simulink model "attitude_filter_wrapper"  (R2023a)
settings: configuration reference "configuration_filter" (kept outside this file)
undefined symbols (not defined in the file): DiscIntNeverNeededParam, Eul_rad, filt, mode, rot_K_est_OB_B_radDs, rot_K_meas_IB_B_radDs, sfor_est_B_mDs, sfor_meas_B_mDs2, sim, x_est
libraries: lib_kinematics x5
settings Model: Creator=FC_dev1  LastModifiedBy=FC_dev1
settings ConfigSetRef: SourceName=configuration_filter  SourceLocation=Base Workspace

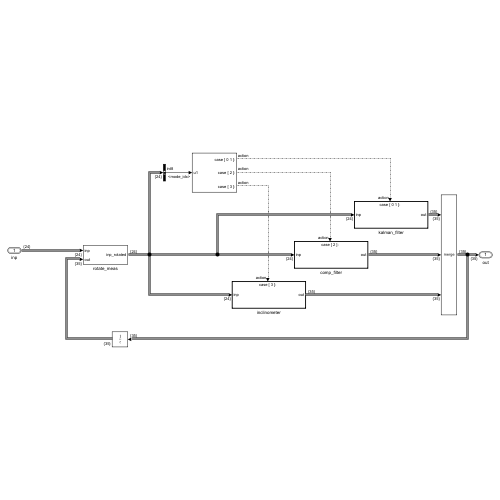
[thumbnail: Simulink's stored preview of the top-level diagram]
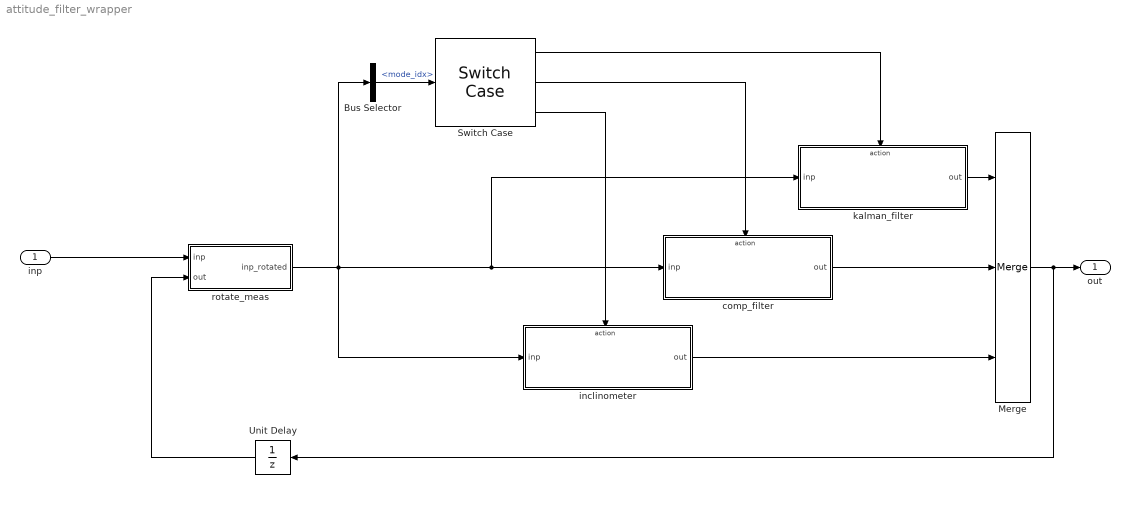
== system attitude_filter_wrapper ==
  inp : Inport  OutDataTypeStr=Bus: inp_Bus
  Bus Selector : BusSelector  OutputSignals=mode_idx
  Merge : Merge  Inputs=3
  Switch Case : SwitchCase  CaseConditions={[filt.modes.kalman_filter, filt.modes.dead_reckoning], filt.modes.comp_filter, filt.modes.inclinometer}  ShowDefaultCase=off
  Unit Delay : UnitDelay  SampleTime=-1  HasFrameUpgradeWarning=on
  comp_filter : Subsystem
  inclinometer : Subsystem
  kalman_filter : Subsystem
  rotate_meas : Subsystem
  out : Outport  OutDataTypeStr=Bus: out_Bus
  wires:
  inp/1 -> rotate_meas/1(inp)
  comp_filter/1(out) -> Merge/2
  Bus Selector/1 -> Switch Case/1  "<mode_idx>"
  Switch Case/1 -> kalman_filter/Action
  Switch Case/2 -> comp_filter/Action
  kalman_filter/1(out) -> Merge/1
  Merge/1 -> Unit Delay/1, out/1
  inclinometer/1(out) -> Merge/3
  Switch Case/3 -> inclinometer/Action
  Unit Delay/1 -> rotate_meas/2(out)
  rotate_meas/1(inp_rotated) -> inclinometer/1(inp), comp_filter/1(inp), kalman_filter/1(inp), Bus Selector/1

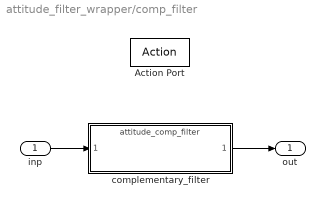
== system attitude_filter_wrapper/comp_filter ==
  inp : Inport  OutDataTypeStr=Bus: inp_Bus
  Action Port : ActionPort  InitializeStates=reset  ActionPortLabel=case [ 2 ]:
  complementary_filter : ModelReference  ModelNameDialog=attitude_comp_filter.slx  SimulationMode=Normal  ModelReferenceVersion=1.231
  out : Outport  OutDataTypeStr=Bus: out_Bus
  wires:
  inp/1 -> complementary_filter/1
  complementary_filter/1 -> out/1

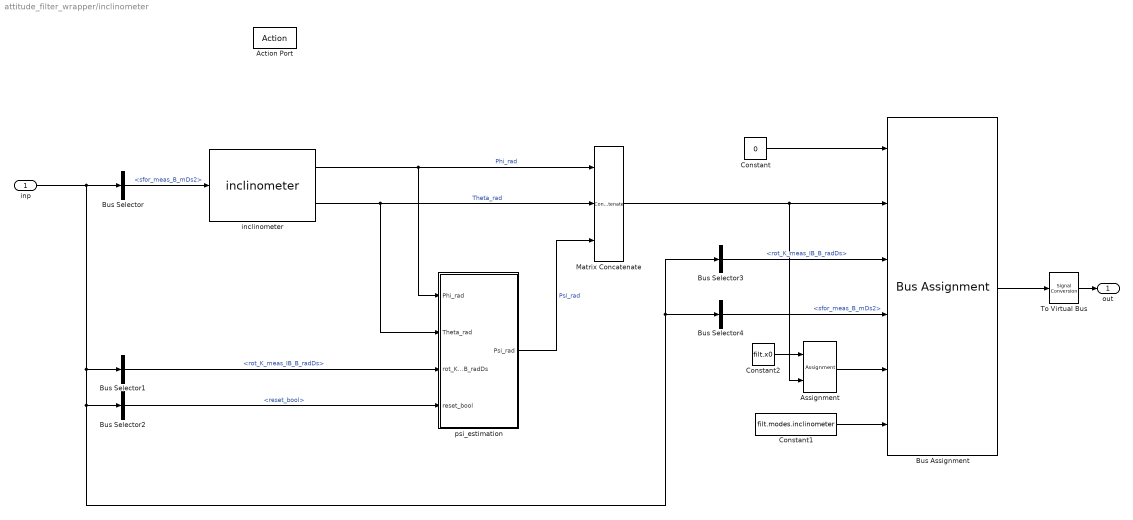
== system attitude_filter_wrapper/inclinometer ==
  inp : Inport  OutDataTypeStr=Bus: inp_Bus
  Action Port : ActionPort  InitializeStates=reset  ActionPortLabel=case [ 3 ]:
  Assignment : Assignment  NumberOfDimensions=2  DiagnosticForDimensions=Warning  IndexOptions=Index vector (dialog),Index vector (dialog)  Indices=filt.eul_idx,1  OutputSizes=1,1
  Bus Assignment : BusAssignment  AssignedSignals=Eul_rad,rot_K_est_OB_B_radDs,sfor_est_B_mDs,x_est,mode
  Bus Selector : BusSelector  OutputSignals=sfor_meas_B_mDs2
  Bus Selector1 : BusSelector  OutputSignals=rot_K_meas_IB_B_radDs
  Bus Selector2 : BusSelector  OutputSignals=reset_bool
  Bus Selector3 : BusSelector  OutputSignals=rot_K_meas_IB_B_radDs
  Bus Selector4 : BusSelector  OutputSignals=sfor_meas_B_mDs2
  Constant : Constant  Value=0  OutDataTypeStr=Bus: out_Bus
  Constant1 : Constant  Value=filt.modes.inclinometer
  Constant2 : Constant  Value=filt.x0  VectorParams1D=off
  Matrix Concatenate : Concatenate  NumInputs=3  Mode=Multidimensional array
  To Virtual Bus : SignalConversion  ConversionOutput=Virtual bus  OverrideOpt=off
  inclinometer : lib_kinematics/inclinometer  SystemSampleTime=-1  VariantActivationTime=update diagram  Latency=0  AutoFrameSizeCalculation=off
  psi_estimation : Subsystem
  out : Outport  OutDataTypeStr=Bus: out_Bus
  wires:
  inp/1 -> Bus Selector4/1, Bus Selector3/1, Bus Selector2/1, Bus Selector1/1, Bus Selector/1
  Bus Selector/1 -> inclinometer/1  "<sfor_meas_B_mDs2>"
  inclinometer/1 -> psi_estimation/1(Phi_rad), Matrix Concatenate/1  "Phi_rad"
  inclinometer/2 -> psi_estimation/2(Theta_rad), Matrix Concatenate/2  "Theta_rad"
  Bus Selector2/1 -> psi_estimation/4(reset_bool)  "<reset_bool>"
  Bus Selector1/1 -> psi_estimation/3(rot_K_OB_B_radDs)  "<rot_K_meas_IB_B_radDs>"
  Constant/1 -> Bus Assignment/1
  psi_estimation/1(Psi_rad) -> Matrix Concatenate/3  "Psi_rad"
  Matrix Concatenate/1 -> Assignment/2, Bus Assignment/2
  Bus Selector3/1 -> Bus Assignment/3  "<rot_K_meas_IB_B_radDs>"
  Bus Selector4/1 -> Bus Assignment/4  "<sfor_meas_B_mDs2>"
  Bus Assignment/1 -> To Virtual Bus/1
  To Virtual Bus/1 -> out/1
  Constant2/1 -> Assignment/1
  Assignment/1 -> Bus Assignment/5
  Constant1/1 -> Bus Assignment/6

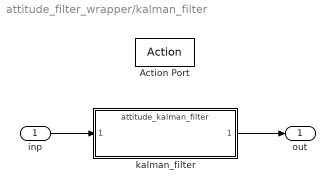
== system attitude_filter_wrapper/kalman_filter ==
  inp : Inport  OutDataTypeStr=Bus: inp_Bus
  Action Port : ActionPort  InitializeStates=reset  ActionPortLabel=case [ 0 1 ]:
  kalman_filter : ModelReference  ModelNameDialog=attitude_kalman_filter.slx  SimulationMode=Normal  ModelReferenceVersion=1.354
  out : Outport  OutDataTypeStr=Bus: out_Bus
  wires:
  inp/1 -> kalman_filter/1
  kalman_filter/1 -> out/1

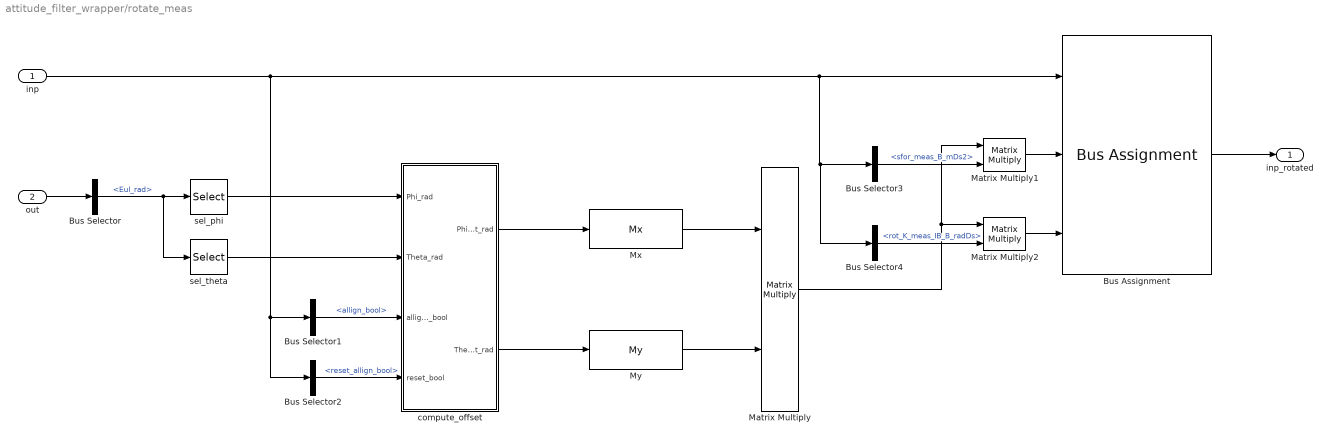
== system attitude_filter_wrapper/rotate_meas ==
  inp : Inport  OutDataTypeStr=Bus: inp_Bus
  out : Inport  Port=2  OutDataTypeStr=Bus: out_Bus
  Bus Assignment : BusAssignment  AssignedSignals=sfor_meas_B_mDs2,rot_K_meas_IB_B_radDs
  Bus Selector : BusSelector  OutputSignals=Eul_rad
  Bus Selector1 : BusSelector  OutputSignals=allign_bool
  Bus Selector2 : BusSelector  OutputSignals=reset_allign_bool
  Bus Selector3 : BusSelector  OutputSignals=sfor_meas_B_mDs2
  Bus Selector4 : BusSelector  OutputSignals=rot_K_meas_IB_B_radDs
  Matrix Multiply : Product  Multiplication=Matrix(*)
  Matrix Multiply1 : Product  Multiplication=Matrix(*)
  Matrix Multiply2 : Product  Multiplication=Matrix(*)
  Mx : lib_kinematics/Mx  SystemSampleTime=-1  VariantActivationTime=update diagram  Latency=0  AutoFrameSizeCalculation=off
  My : lib_kinematics/My  SystemSampleTime=-1  VariantActivationTime=update diagram  Latency=0  AutoFrameSizeCalculation=off
  compute_offset : Subsystem
  sel_phi : Selector  NumberOfDimensions=2  InputPortWidth=3  IndexOptions=Index vector (dialog),Index vector (dialog)  Indices=1,1  OutputSizes=1,1
  sel_theta : Selector  NumberOfDimensions=2  InputPortWidth=3  IndexOptions=Index vector (dialog),Index vector (dialog)  Indices=2,1  OutputSizes=1,1
  inp_rotated : Outport  OutDataTypeStr=Bus: inp_Bus
  wires:
  inp/1 -> Bus Selector2/1, Bus Selector1/1, Bus Selector4/1, Bus Selector3/1, Bus Assignment/1
  out/1 -> Bus Selector/1
  Bus Selector/1 -> sel_theta/1, sel_phi/1  "<Eul_rad>"
  sel_phi/1 -> compute_offset/1(Phi_rad)
  sel_theta/1 -> compute_offset/2(Theta_rad)
  Bus Selector1/1 -> compute_offset/3(allign_bool)  "<allign_bool>"
  Bus Selector2/1 -> compute_offset/4(reset_bool)  "<reset_allign_bool>"
  compute_offset/1(Phi_offset_rad) -> Mx/1
  compute_offset/2(Theta_offset_rad) -> My/1
  Mx/1 -> Matrix Multiply/1
  My/1 -> Matrix Multiply/2
  Bus Assignment/1 -> inp_rotated/1
  Matrix Multiply1/1 -> Bus Assignment/2
  Matrix Multiply/1 -> Matrix Multiply2/1, Matrix Multiply1/1
  Matrix Multiply2/1 -> Bus Assignment/3
  Bus Selector3/1 -> Matrix Multiply1/2  "<sfor_meas_B_mDs2>"
  Bus Selector4/1 -> Matrix Multiply2/2  "<rot_K_meas_IB_B_radDs>"

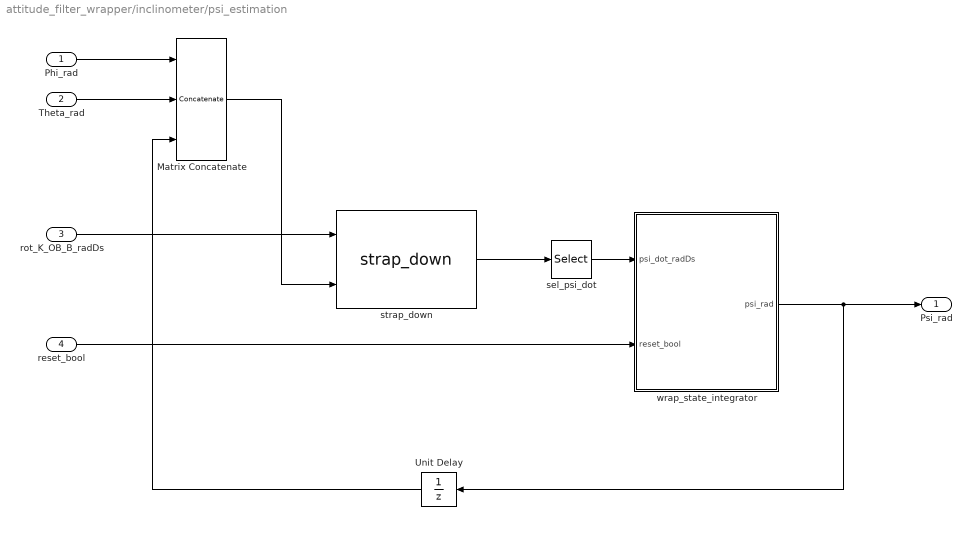
== system attitude_filter_wrapper/inclinometer/psi_estimation ==
  Phi_rad : Inport
  Theta_rad : Inport  Port=2
  rot_K_OB_B_radDs : Inport  Port=3  OutDataTypeStr=single  PortDimensions=[3 1]
  reset_bool : Inport  Port=4
  Matrix Concatenate : Concatenate  NumInputs=3  Mode=Multidimensional array
  Unit Delay : UnitDelay  SampleTime=-1  HasFrameUpgradeWarning=on
  sel_psi_dot : Selector  NumberOfDimensions=2  InputPortWidth=3  IndexOptions=Index vector (dialog),Index vector (dialog)  Indices=3,1  OutputSizes=1,1
  strap_down : lib_kinematics/strap_down  SystemSampleTime=-1  VariantActivationTime=update diagram  Latency=0  AutoFrameSizeCalculation=off
  wrap_state_integrator : Subsystem
  Psi_rad : Outport
  wires:
  rot_K_OB_B_radDs/1 -> strap_down/1
  sel_psi_dot/1 -> wrap_state_integrator/1(psi_dot_radDs)
  strap_down/1 -> sel_psi_dot/1
  wrap_state_integrator/1(psi_rad) -> Unit Delay/1, Psi_rad/1
  reset_bool/1 -> wrap_state_integrator/2(reset_bool)
  Phi_rad/1 -> Matrix Concatenate/1
  Theta_rad/1 -> Matrix Concatenate/2
  Matrix Concatenate/1 -> strap_down/2
  Unit Delay/1 -> Matrix Concatenate/3

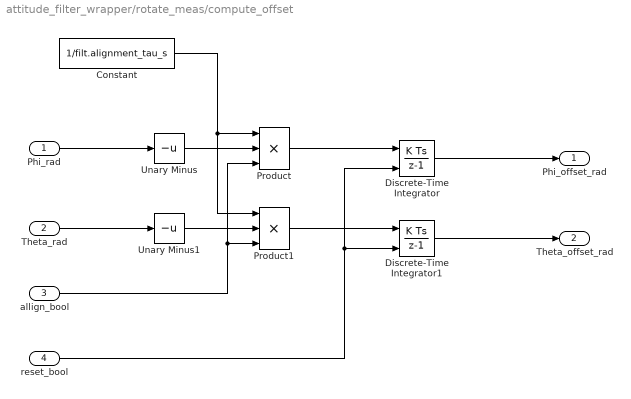
== system attitude_filter_wrapper/rotate_meas/compute_offset ==
  Phi_rad : Inport
  Theta_rad : Inport  Port=2
  allign_bool : Inport  Port=3
  reset_bool : Inport  Port=4
  Constant : Constant  Value=1/filt.alignment_tau_s
  Discrete-Time Integrator : DiscreteIntegrator  ExternalReset=level  SampleTime=sim.sample_time_s  ICPrevOutput=DiscIntNeverNeededParam  ICPrevScaledInput=DiscIntNeverNeededParam
  Discrete-Time Integrator1 : DiscreteIntegrator  ExternalReset=level  SampleTime=sim.sample_time_s  ICPrevOutput=DiscIntNeverNeededParam  ICPrevScaledInput=DiscIntNeverNeededParam
  Product : Product  Inputs=3
  Product1 : Product  Inputs=3
  Unary Minus : UnaryMinus
  Unary Minus1 : UnaryMinus
  Phi_offset_rad : Outport
  Theta_offset_rad : Outport  Port=2
  wires:
  Phi_rad/1 -> Unary Minus/1
  Theta_rad/1 -> Unary Minus1/1
  Unary Minus/1 -> Product/2
  Unary Minus1/1 -> Product1/2
  Constant/1 -> Product1/1, Product/1
  Product/1 -> Discrete-Time Integrator/1
  Product1/1 -> Discrete-Time Integrator1/1
  allign_bool/1 -> Product/3, Product1/3
  reset_bool/1 -> Discrete-Time Integrator/2, Discrete-Time Integrator1/2
  Discrete-Time Integrator/1 -> Phi_offset_rad/1
  Discrete-Time Integrator1/1 -> Theta_offset_rad/1

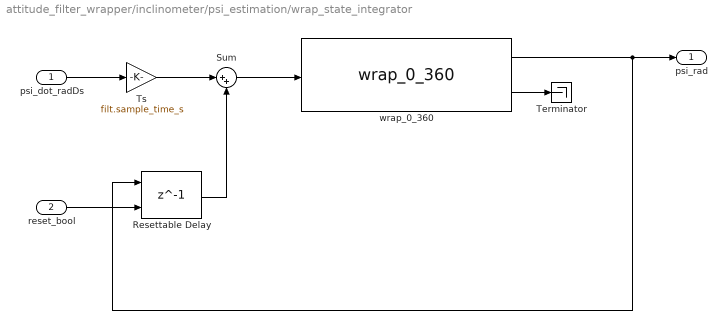
== system attitude_filter_wrapper/inclinometer/psi_estimation/wrap_state_integrator ==
  psi_dot_radDs : Inport
  reset_bool : Inport  Port=2
  Resettable Delay : Delay  DelayLength=1  InitialCondition=0  ExternalReset=Level
      settings: InputPortMap=u0,r5
  Sum : Sum  Inputs=|++
  Terminator : Terminator
  Ts : Gain  Gain=filt.sample_time_s
  wrap_0_360 : lib_kinematics/wrap_0_360  SystemSampleTime=-1  VariantActivationTime=update diagram  Latency=0  AutoFrameSizeCalculation=off
  psi_rad : Outport
  wires:
  psi_dot_radDs/1 -> Ts/1
  Sum/1 -> wrap_0_360/1
  wrap_0_360/1 -> Resettable Delay/1, psi_rad/1
  Ts/1 -> Sum/1
  wrap_0_360/2 -> Terminator/1
  Resettable Delay/1 -> Sum/2
  reset_bool/1 -> Resettable Delay/2
